simulink model "part2"  (R2018b)
settings: Solver=VariableStepAuto  StartTime=0.0  StopTime=2  RelTol=1e-3
libraries: simulink x1
settings Model: Creator=lisazaher  LastModifiedBy=lisazaher

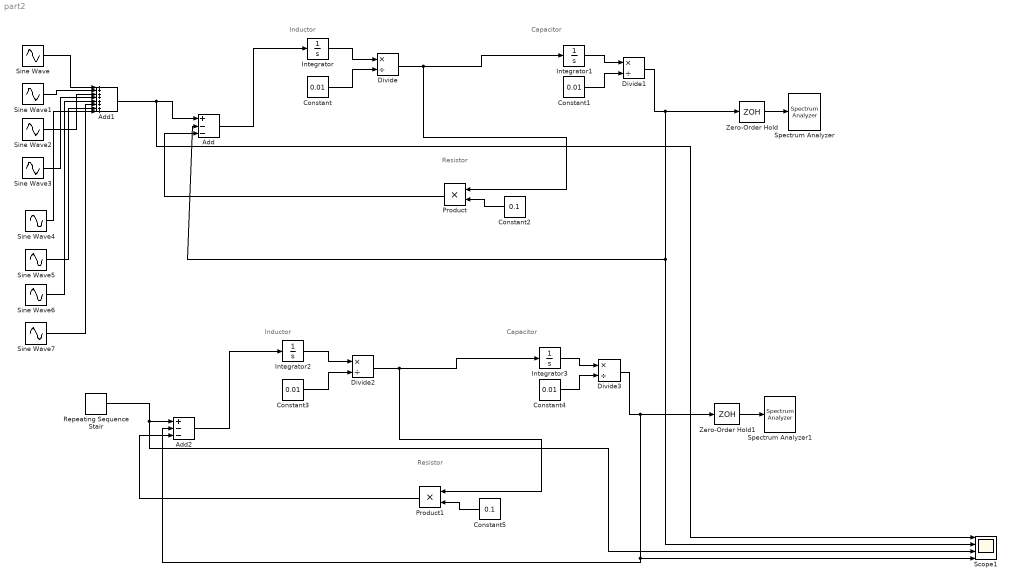
== system part2 ==
  note: Capacitor
  note: Inductor
  note: Resistor
  note: Capacitor
  note: Inductor
  note: Resistor
  Add : Sum  Inputs=+--
  Add1 : Sum  Inputs=++++++++
  Add2 : Sum  Inputs=+--
  Constant{,1,3..4} (4 alike) : Constant  Value=0.01
  Constant2 : Constant  Value=0.1
  Constant5 : Constant  Value=0.1
  Divide{,1..3} (4 alike) : Product  Inputs=*/
  Integrator : Integrator
  Integrator1 : Integrator  InitialCondition=0.0
  Integrator2 : Integrator
  Integrator3 : Integrator  InitialCondition=0.0
  Product : Product
  Product1 : Product
  Repeating Sequence Stair : simulink/Sources/Repeating Sequence Stair  OutValues=[1 -1].'  tsamp=1/64  OutMin=-1  OutMax=1  OutDataTypeStr=double  OutputDataTypeScalingMode=double  OutDataType=fixdt(0,8)  ConRadixGroup=Best Precision: Vector-wise  OutScaling=2^-12
  Scope1 : Scope  NumInputPorts=4
  Sine Wave : Sin  Amplitude=4/pi  Frequency=64*pi  SampleTime=0
  Sine Wave1 : Sin  Amplitude=4/(3*pi)  Frequency=6*32*pi  SampleTime=0
  Sine Wave2 : Sin  Amplitude=4/(5*pi)  Frequency=10*pi*32  SampleTime=0
  Sine Wave3 : Sin  Amplitude=4/(7*pi)  Frequency=14*pi*32  SampleTime=0
  Sine Wave4 : Sin  Amplitude=4/(9*pi)  Frequency=32*18*pi  SampleTime=0
  Sine Wave5 : Sin  Amplitude=4/(11*pi)  Frequency=22*32*pi  SampleTime=0
  Sine Wave6 : Sin  Amplitude=4/(13*pi)  Frequency=26*pi*32  SampleTime=0
  Sine Wave7 : Sin  Amplitude=4/(15*pi)  Frequency=30*pi*32  SampleTime=0
  Spectrum Analyzer : SpectrumAnalyzer
  Spectrum Analyzer1 : SpectrumAnalyzer
  Zero-Order Hold : ZeroOrderHold  SampleTime=2^-10
  Zero-Order Hold1 : ZeroOrderHold  SampleTime=2^-10
  wires:
  Constant/1 -> Divide/2
  Constant1/1 -> Divide1/2
  Divide/1 -> Product/1, Integrator1/1
  Product/1 -> Add/3
  Constant2/1 -> Product/2
  Integrator/1 -> Divide/1
  Integrator1/1 -> Divide1/1
  Divide1/1 -> Zero-Order Hold/1, Scope1/2, Add/2
  Zero-Order Hold/1 -> Spectrum Analyzer/1
  Add/1 -> Integrator/1
  Add1/1 -> Scope1/1, Add/1
  Add2/1 -> Integrator2/1
  Product1/1 -> Add2/3
  Constant3/1 -> Divide2/2
  Constant4/1 -> Divide3/2
  Divide3/1 -> Zero-Order Hold1/1, Scope1/4, Add2/2
  Repeating Sequence Stair/1 -> Scope1/3, Add2/1
  Divide2/1 -> Product1/1, Integrator3/1
  Zero-Order Hold1/1 -> Spectrum Analyzer1/1
  Constant5/1 -> Product1/2
  Integrator2/1 -> Divide2/1
  Integrator3/1 -> Divide3/1
  Sine Wave7/1 -> Add1/6
  Sine Wave6/1 -> Add1/5
  Sine Wave5/1 -> Add1/7
  Sine Wave1/1 -> Add1/2
  Sine Wave3/1 -> Add1/4
  Sine Wave4/1 -> Add1/8
  Sine Wave/1 -> Add1/1
  Sine Wave2/1 -> Add1/3
